simulink model "streamSignalEmulation2"  (R2013b)
settings: Solver=VariableStepDiscrete  StartTime=0.0  StopTime=30  FixedStep=1e-3  MaxStep=100e-3  RelTol=1e-3
undefined symbols (not defined in the file or in its folder): sigbuilder_block
libraries: simulink x8, powerlib_meascontrol x2
settings Model: PauseTimes=1.8  NumberOfSteps=100  SnapshotBufferSize=10000  SnapshotInterval=100  Creator=mainster  LastModifiedBy=mainster

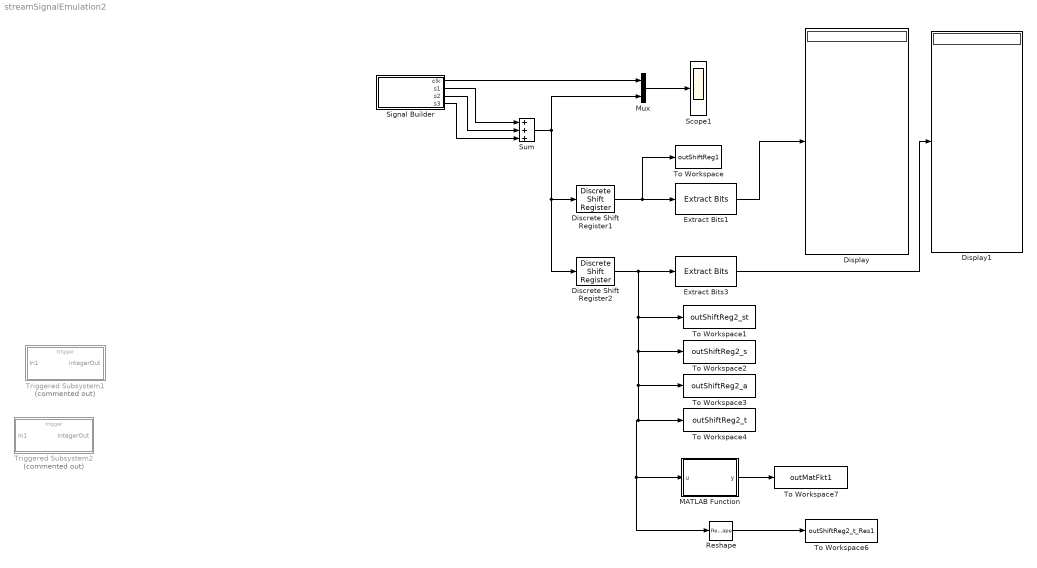
== system streamSignalEmulation2 ==
  Discrete Shift Register1 : powerlib_meascontrol/Additional Components/Discrete Shift Register  NSamples=16  InitialValue=0  Ts=1
  Discrete Shift Register2 : powerlib_meascontrol/Additional Components/Discrete Shift Register  NSamples=16  InitialValue=0  Ts=2
  Display : Display
      settings: Format=binary (Stored Integer)
  Display1 : Display
      settings: Format=binary (Stored Integer)
  Extract Bits1 : simulink/Logic and Bit Operations/Extract Bits  bitsToExtract=Range of bits  numBits=8  bitIdxRange=[0 17]  outScalingMode=Treat bit field as an integer
  Extract Bits3 : simulink/Logic and Bit Operations/Extract Bits  bitsToExtract=Range of bits  numBits=8  bitIdxRange=[0 17]  outScalingMode=Treat bit field as an integer
  MATLAB Function : MATLAB Function  TreatAsAtomicUnit=on
  Mux : Mux  Inputs=2
  Reshape : Reshape  OutputDimensionality=Customize  OutputDimensions=[1,16]
  Scope1 : Scope
      settings: ShowLegends=on  TimeRange=30  YMin=-0.2  YMax=2.2
  Signal Builder : Subsystem  Tag=STV Subsys  LoadFcn=sigbuilder_block('load',[4.5 57.75 837.75 399.75 ]);  StartFcn=sigbuilder_block('start');  StopFcn=sigbuilder_block('stop');  ClipboardFcn=sigbuilder_block('clipboard');  mask(Sigbuilder block){}
      mask help: Simulink:masks:SigbuilderBlock_MD
      mask init:
      | if ~strcmp(get_param(bdroot(gcbh),'SimulationStatus'),'stopped') tuvar = sigbuilder_block('maskInit'); end
      settings: CopyFcn=sigbuilder_block('copy');  DeleteFcn=sigbuilder_block('delete');  ModelCloseFcn=sigbuilder_block('modelClose');  PreSaveFcn=sigbuilder_block('preSave');  PauseFcn=sigbuilder_block('pause');  ContinueFcn=sigbuilder_block('continue');  NameChangeFcn=sigbuilder_block('namechange');  OpenFcn=sigbuilder_block('open',[434.25 88.5 837.75 399.75 ]);  CloseFcn=sigbuilder_block('close');
      mask Display: plot(0, 0, 100, 100,[2, 2, 32, 32, 2], [68, 8, 8, 68, 68],[32, 2], [38, 38], [32, 19, 2],[53, 60, 44], [32, 17, 17, 2],[16, 16, 31, 31]);txt = getActiveGroup(gcbh);text(2, 100, txt,'verticalAlignment', 'top');
  Sum : Sum  Inputs=+++
  To Workspace : ToWorkspace  VariableName=outShiftReg1  SampleTime=-1  SaveFormat=Structure
  To Workspace1 : ToWorkspace  VariableName=outShiftReg2_st  SampleTime=-1  SaveFormat=Structure With Time
  To Workspace2 : ToWorkspace  VariableName=outShiftReg2_s  SampleTime=-1  SaveFormat=Structure
  To Workspace3 : ToWorkspace  VariableName=outShiftReg2_a  SampleTime=-1
  To Workspace4 : ToWorkspace  VariableName=outShiftReg2_t  SampleTime=-1  SaveFormat=Timeseries
  To Workspace6 : ToWorkspace  VariableName=outShiftReg2_t_Res1  SampleTime=-1  SaveFormat=Timeseries
  To Workspace7 : ToWorkspace  VariableName=outMatFkt1  SampleTime=-1  SaveFormat=Timeseries
  Triggered Subsystem1 : Subsystem  Commented=on  TreatAsAtomicUnit=on
  Triggered Subsystem2 : Subsystem  Commented=on  TreatAsAtomicUnit=on
  wires:
  Extract Bits1/1 -> Display/1
  Signal Builder/3(s2) -> Sum/2
  Signal Builder/2(s1) -> Sum/1
  Signal Builder/4(s3) -> Sum/3
  Discrete Shift Register1/1 -> To Workspace/1, Extract Bits1/1
  Extract Bits3/1 -> Display1/1
  Mux/1 -> Scope1/1
  Sum/1 -> Discrete Shift Register1/1, Discrete Shift Register2/1, Mux/2
  Signal Builder/1(clk) -> Mux/1
  Discrete Shift Register2/1 -> To Workspace1/1, To Workspace2/1, To Workspace3/1, MATLAB Function/1(u), Reshape/1, To Workspace4/1, Extract Bits3/1
  Reshape/1 -> To Workspace6/1
  MATLAB Function/1(y) -> To Workspace7/1

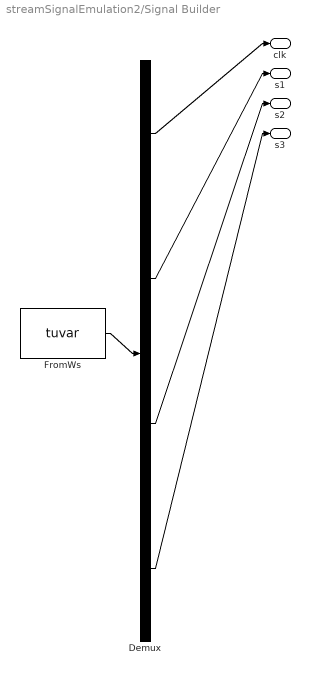
== system streamSignalEmulation2/Signal Builder ==
  Demux : Demux  Tag=STV Demux
  FromWs : FromWorkspace  Tag=STV FromWs  VariableName=tuvar  SampleTime=0
      SigBuilderData=|
      | common.afterFinalStr = 'Extrapolate'
      | common.sampleTime = 0
      | dataSet.timeRange = [0 32]
      | dataSet.name = 'Group 1'
      | sbobj.Groups.Name = 'Group 1'
      | sbobj.Groups.Signals(1).Name = 'clk'
      | sbobj.Groups.Signals(1).XData = [0 1 1 2 2 3 3 4 4 5 5 6 6 7 7 8 8 9 9 10 10 11 11 12 12 13 13 14 14 15 15 16 16 17 17 18 18 19 19 20 20 21 21 22 22 23 23 24 24 25 25 26 26 27 27 28 28 29 29 30 30 31 31 32]
      | sbobj.Groups.Signals(1).YData = [1 1 0 0 1 1 0 0 1 1 0 0 1 1 0 0 1 1 0 0 1 1 0 0 1 1 0 0 1 1 0 0 1 1 0 0 1 1 0 0 1 1 0 0 1 1 0 0 1 1 0 0 1 1 0 0 1 1 0 0 1 1 0 0]
      | sbobj.Groups.Signals(2).Name = 's1'
      | sbobj.Groups.Signals(2).XData = [0 0.5 0.5 1.52 1.52 32]
      | sbobj.Groups.Signals(2).YData = [0 0 1 1 0 0]
      | sbobj.Groups.Signals(3).Name = 's2'
      | sbobj.Groups.Signals(3).XData = [0 6 7.5 7.5 12.5 12.5 32]
      | sbobj.Groups.Signals(3).YData = [0 0 0 1 1 0 0]
      | sbobj.Groups.Signals(4).Name = 's3'
      | sbobj.Groups.Signals(4).XData = [0 17.5 17.5 29.5 29.5 32]
      | sbobj.Groups.Signals(4).YData = [0 0 1 1 0 0]
      | sbobj.Groups.TimeRange = [0 0.032]
  clk : Outport  Tag=STV Outport
  s1 : Outport  Tag=STV Outport  Port=2
  s2 : Outport  Tag=STV Outport  Port=3
  s3 : Outport  Tag=STV Outport  Port=4
  wires:
  FromWs/1 -> Demux/1
  Demux/1 -> clk/1
  Demux/2 -> s1/1
  Demux/3 -> s2/1
  Demux/4 -> s3/1

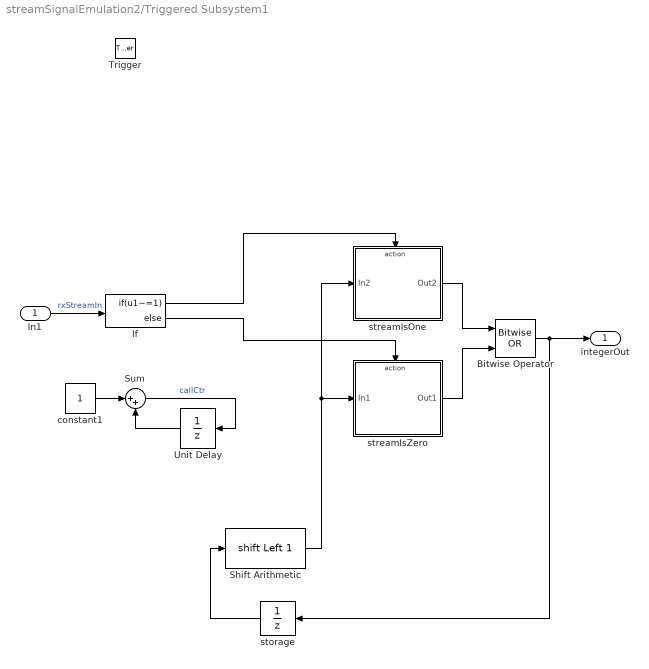
== system streamSignalEmulation2/Triggered Subsystem1 ==
  In1 : Inport
  Trigger : TriggerPort  TriggerType=falling
  Bitwise Operator : simulink/Logic and Bit Operations/Bitwise Operator  logicop=OR  UseBitMask=off  NumInputPorts=2  BitMask=bin2dec('11011001')  BitMaskRealWorld=Stored Integer
  If : If  IfExpression=u1~=1
  Shift Arithmetic : ArithShift  BitShiftNumber=1  BitShiftDirection=Left  DiagnosticForOORShift=Warning  CheckOORBitShift=on
  Sum : Sum  Inputs=|++  SaturateOnIntegerOverflow=on  InputSameDT=on  OutDataTypeStr=Inherit: Same as first input
  Unit Delay : UnitDelay  SampleTime=-1
  constant1 : Constant  OutDataTypeStr=int8  LockScale=on
  storage : UnitDelay  SampleTime=-1
  streamIsOne : Subsystem  TreatAsAtomicUnit=on
  streamIsZero : Subsystem  TreatAsAtomicUnit=on
  integerOut : Outport
  wires:
  In1/1 -> If/1  "rxStreamIn"
  Sum/1 -> Unit Delay/1  "callCtr"
  constant1/1 -> Sum/1
  Unit Delay/1 -> Sum/2
  Shift Arithmetic/1 -> streamIsOne/1(In2), streamIsZero/1(In1)
  storage/1 -> Shift Arithmetic/1
  If/2 -> streamIsZero/Action
  If/1 -> streamIsOne/Action
  streamIsOne/1(Out2) -> Bitwise Operator/1
  streamIsZero/1(Out1) -> Bitwise Operator/2
  Bitwise Operator/1 -> integerOut/1, storage/1

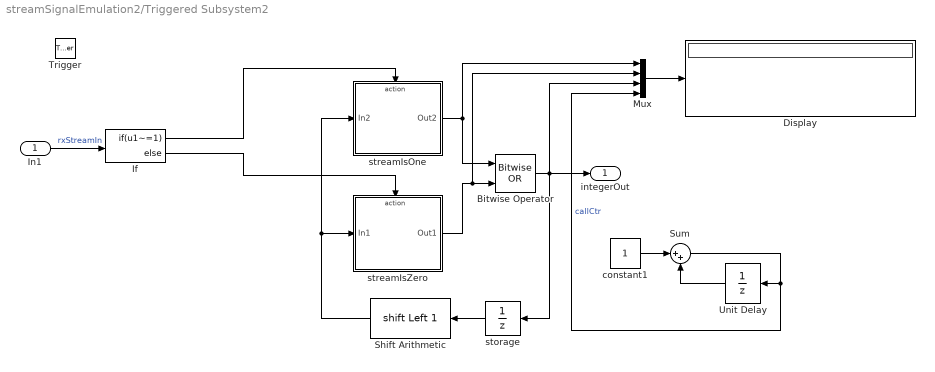
== system streamSignalEmulation2/Triggered Subsystem2 ==
  In1 : Inport
  Trigger : TriggerPort  TriggerType=falling
  Bitwise Operator : simulink/Logic and Bit Operations/Bitwise Operator  logicop=OR  UseBitMask=off  NumInputPorts=2  BitMask=bin2dec('11011001')  BitMaskRealWorld=Stored Integer
  Display : Display
      settings: Format=binary (Stored Integer)
  If : If  IfExpression=u1~=1
  Mux : Mux
  Shift Arithmetic : ArithShift  BitShiftNumber=1  BitShiftDirection=Left  DiagnosticForOORShift=Warning  CheckOORBitShift=on
  Sum : Sum  Inputs=|++  SaturateOnIntegerOverflow=on  InputSameDT=on  OutDataTypeStr=Inherit: Same as first input
  Unit Delay : UnitDelay  SampleTime=-1
  constant1 : Constant  OutDataTypeStr=uint32  LockScale=on
  storage : UnitDelay  SampleTime=-1
  streamIsOne : Subsystem  TreatAsAtomicUnit=on
  streamIsZero : Subsystem  TreatAsAtomicUnit=on
  integerOut : Outport
  wires:
  In1/1 -> If/1  "rxStreamIn"
  Sum/1 -> Mux/4, Unit Delay/1  "callCtr"
  constant1/1 -> Sum/1
  Unit Delay/1 -> Sum/2
  Shift Arithmetic/1 -> streamIsOne/1(In2), streamIsZero/1(In1)
  storage/1 -> Shift Arithmetic/1
  If/2 -> streamIsZero/Action
  If/1 -> streamIsOne/Action
  streamIsOne/1(Out2) -> Bitwise Operator/1, Mux/1
  streamIsZero/1(Out1) -> Mux/2, Bitwise Operator/2
  Bitwise Operator/1 -> Mux/3, integerOut/1, storage/1
  Mux/1 -> Display/1

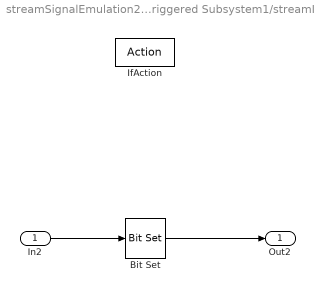
== system streamSignalEmulation2/Triggered Subsystem1/streamIsOne ==
  In2 : Inport  OutDataTypeStr=uint8
  IfAction : ActionPort
  Bit Set : simulink/Logic and Bit Operations/Bit Set  iBit=0
  Out2 : Outport  OutDataTypeStr=uint8
  wires:
  In2/1 -> Bit Set/1
  Bit Set/1 -> Out2/1

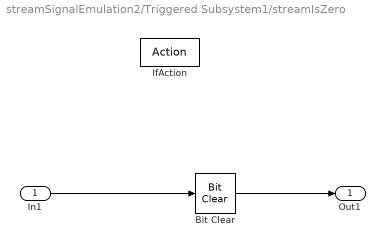
== system streamSignalEmulation2/Triggered Subsystem1/streamIsZero ==
  In1 : Inport  OutDataTypeStr=uint8
  IfAction : ActionPort
  Bit Clear : simulink/Logic and Bit Operations/Bit Clear  iBit=0
  Out1 : Outport  OutDataTypeStr=uint8
  wires:
  In1/1 -> Bit Clear/1
  Bit Clear/1 -> Out1/1

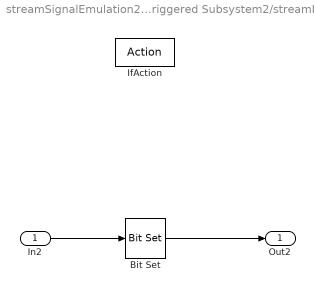
== system streamSignalEmulation2/Triggered Subsystem2/streamIsOne ==
  In2 : Inport  OutDataTypeStr=uint32
  IfAction : ActionPort
  Bit Set : simulink/Logic and Bit Operations/Bit Set  iBit=0
  Out2 : Outport
  wires:
  In2/1 -> Bit Set/1
  Bit Set/1 -> Out2/1

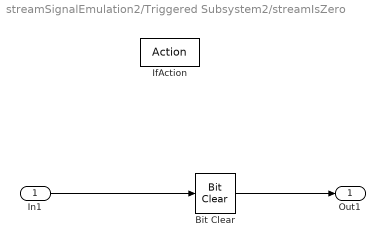
== system streamSignalEmulation2/Triggered Subsystem2/streamIsZero ==
  In1 : Inport  OutDataTypeStr=uint32
  IfAction : ActionPort
  Bit Clear : simulink/Logic and Bit Operations/Bit Clear  iBit=0
  Out1 : Outport  OutDataTypeStr=uint32  LockScale=on
  wires:
  In1/1 -> Bit Clear/1
  Bit Clear/1 -> Out1/1

== matlab function streamSignalEmulation2/MATLAB Function ==
  data: u input; y output
function y = fcn(u)
%#codegen
%exp1=u.signals.values;
%y=[1:16];

y = u(1,1:end);
